simulink model "Biodigestor_3"  (R2017b)
settings: Solver=VariableStepAuto  StartTime=0  StopTime=168  RelTol=1e-3  EnableMultiTasking=on
settings Model: Creator=yoga 500  LastModifiedBy=yoga 500
settings DataIOCC: LimitDataPoints=on  MaxDataPoints=1000000  SaveFormat=Array  SignalLoggingSaveFormat=ModelDataLogs  SignalLoggingName=sigsOut
settings DebuggingCC: SaveWithParameterizedLinksMsg=none  UnderspecifiedInitializationDetection=Classic  MergeDetectMultiDrivingBlocksExec=none  SignalResolutionControl=TryResolveAllWithWarning  MultiTaskDSMMsg=warning  MultiTaskCondExecSysMsg=none
settings HardwareCC: ProdBitPerPointer=32  ProdBitPerSizeT=32  ProdBitPerPtrDiffT=32  ProdLargestAtomicFloat=None  ProdIntDivRoundTo=Undefined  ProdEndianess=Unspecified  ProdWordSize=32  ProdHWDeviceType=32-bit Generic  TargetUnknown=on
settings ModelReferenceCC: PropagateSignalLabelsOutOfModel=off
settings CodeAppCC: StateflowObjectComments=on
settings GRTTargetCC: TargetLangStandard=C89/C90 (ANSI)  CombineOutputUpdateFcns=off  GRTInterface=on
settings ConfigComp: CovMetricSettings=dw  CovHtmlReporting=on  CovSaveCumulativeToWorkspaceVar=on  CovSaveSingleToWorkspaceVar=on  CovExternalEMLEnable=off

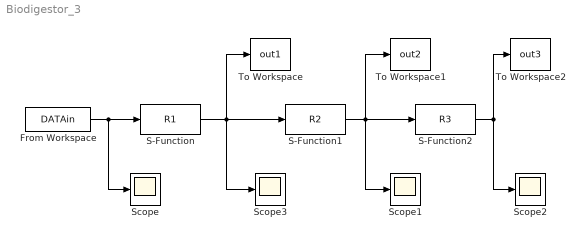
== system Biodigestor_3 ==
  From Workspace : FromWorkspace  VariableName=DATAin  SampleTime=0
  S-Function : S-Function  FunctionName=R1  SFunctionDeploymentMode=off  EnableBusSupport=off
  S-Function1 : S-Function  FunctionName=R2  SFunctionDeploymentMode=off  EnableBusSupport=off
  S-Function2 : S-Function  FunctionName=R3  SFunctionDeploymentMode=off  EnableBusSupport=off
  Scope{,1..3} (4 alike) : Scope
  To Workspace : ToWorkspace  VariableName=out1  SampleTime=-1
  To Workspace1 : ToWorkspace  VariableName=out2  SampleTime=-1
  To Workspace2 : ToWorkspace  VariableName=out3  SampleTime=-1
  wires:
  From Workspace/1 -> Scope/1, S-Function/1
  S-Function/1 -> Scope3/1, To Workspace/1, S-Function1/1
  S-Function1/1 -> S-Function2/1, Scope1/1, To Workspace1/1
  S-Function2/1 -> To Workspace2/1, Scope2/1
